simulink model "spring_mass_tyre_frame"  (R2017b)
settings: Solver=VariableStepAuto  StartTime=0.0  StopTime=92  RelTol=1e-3
undefined symbols (not defined in the file): kt, m
settings Model: Creator=mm395  LastModifiedBy=mm395

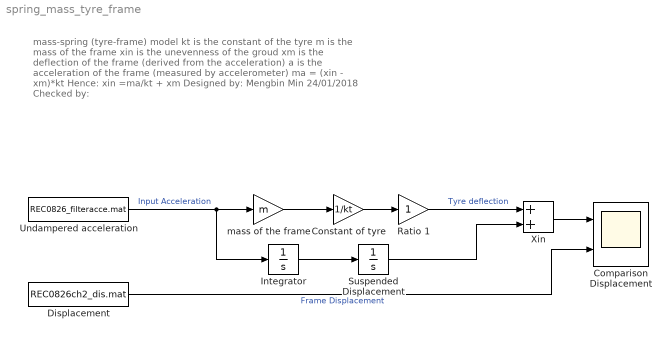
== system spring_mass_tyre_frame ==
  note: mass-spring (tyre-frame) model
      | kt is the constant of the tyre
      | m is the mass of the frame
      | xin is the unevenness of the groud
      | xm is the deflection of the frame (derived from the acceleration)
      | a is the acceleration of the frame (measured by accelerometer)
      |
      | ma = (xin - xm)*kt
      | Hence: xin =ma/kt + xm
      |
      | Designed by: Mengbin Min 24/01/2018
      | Checked by:
  Comparison Displacement : Scope  NumInputPorts=2
  Constant of tyre : Gain  Gain=1/kt
  Displacement : FromFile  FileName=REC0826ch2_dis.mat  SampleTime=1/3200  ExtrapolationBeforeFirstDataPoint=Hold first value  ExtrapolationAfterLastDataPoint=Hold last value
  Integrator : Integrator
  Ratio 1 : Gain
  Suspended Displacement : Integrator
  Undampered acceleration : FromFile  FileName=REC0826_filteracce.mat  SampleTime=1/3200  ExtrapolationBeforeFirstDataPoint=Hold first value  ExtrapolationAfterLastDataPoint=Hold last value
  Xin : Sum
  mass of the frame : Gain  Gain=m
  wires:
  Undampered acceleration/1 -> Integrator/1, mass of the frame/1  "Input Acceleration"
  Ratio 1/1 -> Xin/1  "Tyre deflection"
  Integrator/1 -> Suspended Displacement/1
  Displacement/1 -> Comparison Displacement/2  "Frame Displacement"
  Constant of tyre/1 -> Ratio 1/1
  mass of the frame/1 -> Constant of tyre/1
  Suspended Displacement/1 -> Xin/2
  Xin/1 -> Comparison Displacement/1
